simulink library "oceanFloorContactModel_ul"  (R2020a)
settings: Solver=VariableStepAuto  StartTime=0.0  StopTime=10.0  RelTol=1e-3
undefined symbols (not defined in the file): gndStn
libraries: vrlib x3, eulAng2RotMat_ul x1
settings Model: Creator=mitch  LastModifiedBy=mitch

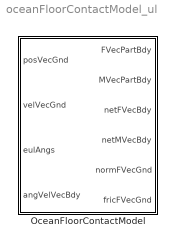
== system oceanFloorContactModel_ul ==
  OceanFloorContactModel : Subsystem  TreatAsAtomicUnit=on  mask{gs=gndStn, momArms=0}
      mask prompts: gs "OCT.floor ocean floor obj"; momArms "Vechicle moment arms"

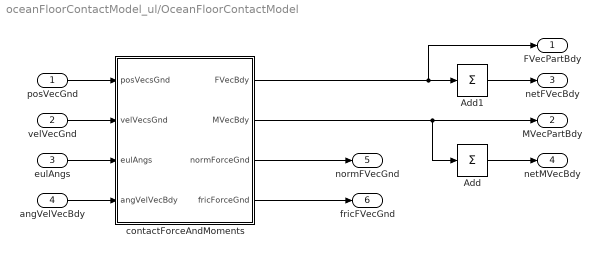
== system oceanFloorContactModel_ul/OceanFloorContactModel ==
  posVecGnd : Inport
  velVecGnd : Inport  Port=2
  eulAngs : Inport  Port=3
  angVelVecBdy : Inport  Port=4
  Add : Sum  Inputs=+  CollapseMode=Specified dimension  CollapseDim=2
  Add1 : Sum  Inputs=+  CollapseMode=Specified dimension  CollapseDim=2
  contactForceAndMoments : Subsystem  mask{z0=gs.bedrockZ.Value, z1=gs.oceanFloorZ.Value, zStar=gs.stiffnessZPt.Value, FStar=gs.stiffnessFMag.Value, mu=gs.fricCoeff.Value, momArmVecs=momArms}
      mask prompts: z0 "Bedrock z Position"; z1 "Ocean floor z Position"; zStar "Stiffness z Point"; FStar "Stiffness Normal Force [N]"; mu "Friction Coeff"; momArmVecs "Mom Arm Vecs Bdy"
  FVecPartBdy : Outport
  MVecPartBdy : Outport  Port=2
  netFVecBdy : Outport  Port=3
  netMVecBdy : Outport  Port=4
  normFVecGnd : Outport  Port=5
  fricFVecGnd : Outport  Port=6
  wires:
  contactForceAndMoments/1(FVecBdy) -> FVecPartBdy/1, Add1/1
  Add/1 -> netMVecBdy/1
  Add1/1 -> netFVecBdy/1
  contactForceAndMoments/2(MVecBdy) -> Add/1, MVecPartBdy/1
  eulAngs/1 -> contactForceAndMoments/3(eulAngs)
  posVecGnd/1 -> contactForceAndMoments/1(posVecsGnd)
  velVecGnd/1 -> contactForceAndMoments/2(velVecsGnd)
  angVelVecBdy/1 -> contactForceAndMoments/4(angVelVecBdy)
  contactForceAndMoments/3(normForceGnd) -> normFVecGnd/1
  contactForceAndMoments/4(fricForceGnd) -> fricFVecGnd/1

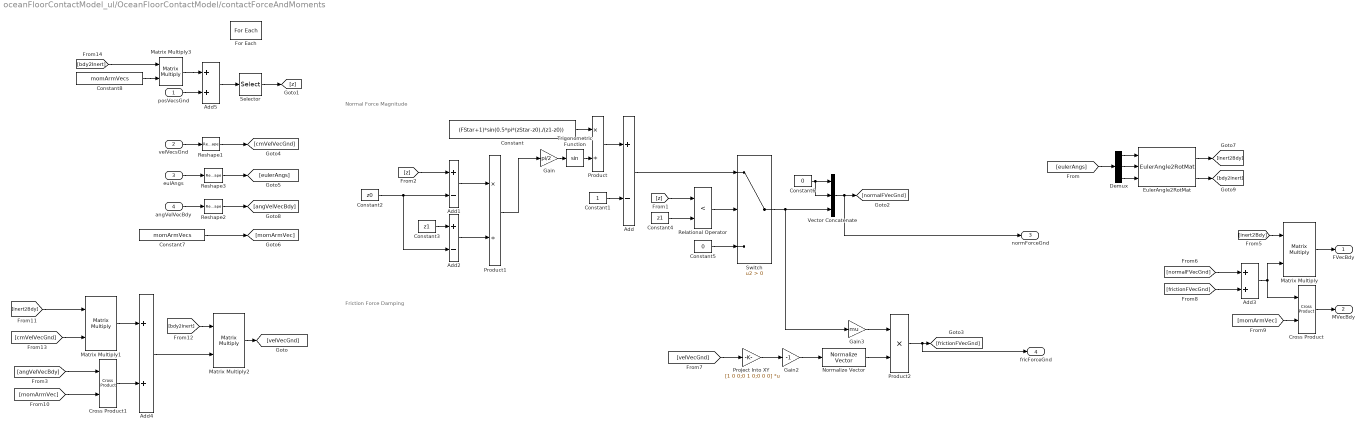
== system oceanFloorContactModel_ul/OceanFloorContactModel/contactForceAndMoments ==
  note: Friction Force Damping
  note: Normal Force Magnitude
  posVecsGnd : Inport  PortDimensions=[3 1]
  velVecsGnd : Inport  Port=2  PortDimensions=[3 1]
  eulAngs : Inport  Port=3  PortDimensions=[3 1]
  angVelVecBdy : Inport  Port=4  PortDimensions=[3 1]
  Add : Sum  Inputs=+-
  Add1 : Sum  Inputs=+-
  Add2 : Sum  Inputs=+-
  Add3 : Sum
  Add4 : Sum
  Add5 : Sum
  Constant : Constant  Value=(FStar+1)*sin(0.5*pi*(zStar-z0)./(z1-z0))
  Constant1 : Constant
  Constant2 : Constant  Value=z0
  Constant3 : Constant  Value=z1
  Constant4 : Constant  Value=z1
  Constant5 : Constant  Value=0
  Constant6 : Constant  Value=0
  Constant7 : Constant  Value=momArmVecs
  Constant8 : Constant  Value=momArmVecs
  Cross Product : vrlib/Utilities/Cross Product
  Cross Product1 : vrlib/Utilities/Cross Product
  Demux : Demux  Outputs=3
  EulerAngle2RotMat : eulAng2RotMat_ul/EulerAngle2RotMat  SystemSampleTime=-1  Latency=0  AutoFrameSizeCalculation=off
  For Each : ForEach  DisableCoverage=on  IterateSubsysMaskParameter=off,off,off,off,off,on  SubsysMaskParameterIterationDimension=1,1,1,1,1,2
  Gain : Gain  Gain=pi/2
  Gain2 : Gain  Gain=-1
  Gain3 : Gain  Gain=mu
  Matrix Multiply{,1..3} (4 alike) : Product  Multiplication=Matrix(*)
  Normalize Vector : vrlib/Utilities/Normalize Vector  maxzero=0
  Product : Product  Inputs=*/
  Product1 : Product  Inputs=*/
  Product2 : Product
  Project Into XY : Gain  Gain=[1 0 0;0 1 0;0 0 0]  Multiplication=Matrix(K*u)
  Relational Operator : RelationalOperator  Operator=<  OutDataTypeStr=boolean  RndMeth=Simplest
  Reshape1 : Reshape  OutputDimensionality=Column vector (2-D)
  Reshape2 : Reshape  OutputDimensionality=Column vector (2-D)
  Reshape3 : Reshape  OutputDimensionality=Column vector (2-D)
  Selector : Selector  InputPortWidth=3  IndexOptions=Index vector (dialog)  Indices=3  OutputSizes=1
  Switch : Switch  Criteria=u2 > Threshold
  Trigonometric Function : Trigonometry
  Vector Concatenate : Concatenate  NumInputs=3
  FVecBdy : Outport  ConcatenationDimension=2
  MVecBdy : Outport  Port=2  ConcatenationDimension=2
  normForceGnd : Outport  Port=3  ConcatenationDimension=2
  fricForceGnd : Outport  Port=4  ConcatenationDimension=2
  wires:
  Constant/1 -> Product/1
  posVecsGnd/1 -> Add5/2
  Product/1 -> Add/1
  Constant1/1 -> Add/2
  Trigonometric Function/1 -> Product/2
  Gain/1 -> Trigonometric Function/1
  Add1/1 -> Product1/1
  Add2/1 -> Product1/2
  Selector/1 -> [z]
  Constant2/1 -> Add2/2, Add1/2
  Constant3/1 -> Add2/1
  Product1/1 -> Gain/1
  Add/1 -> Switch/1
  [z] -> Relational Operator/1
  Constant4/1 -> Relational Operator/2
  Relational Operator/1 -> Switch/2
  [z] -> Add1/1
  Constant5/1 -> Switch/3
  velVecsGnd/1 -> Reshape1/1
  Project Into XY/1 -> Gain2/1
  Gain2/1 -> Normalize Vector/1
  Switch/1 -> Gain3/1, Vector Concatenate/3
  Gain3/1 -> Product2/1
  Normalize Vector/1 -> Product2/2
  Product2/1 -> fricForceGnd/1, [frictionFVecGnd]
  Reshape1/1 -> [cmVelVecGnd]
  [velVecGnd] -> Project Into XY/1
  Constant6/1 -> Vector Concatenate/2, Vector Concatenate/1
  eulAngs/1 -> Reshape3/1
  [eulerAngs] -> Demux/1
  Demux/1 -> EulerAngle2RotMat/1
  Demux/2 -> EulerAngle2RotMat/2
  Demux/3 -> EulerAngle2RotMat/3
  EulerAngle2RotMat/2 -> [bdy2Inert]
  EulerAngle2RotMat/1 -> [inert2Bdy]
  [normalFVecGnd] -> Add3/1
  [frictionFVecGnd] -> Add3/2
  Add3/1 -> Matrix Multiply/2, Cross Product/1
  Matrix Multiply/1 -> FVecBdy/1
  [inert2Bdy] -> Matrix Multiply/1
  Cross Product/1 -> MVecBdy/1
  [momArmVec] -> Cross Product/2
  Constant7/1 -> [momArmVec]
  angVelVecBdy/1 -> Reshape2/1
  Reshape2/1 -> [angVelVecBdy]
  Reshape3/1 -> [eulerAngs]
  [angVelVecBdy] -> Cross Product1/1
  [momArmVec] -> Cross Product1/2
  Cross Product1/1 -> Add4/2
  Add4/1 -> Matrix Multiply2/2
  [cmVelVecGnd] -> Matrix Multiply1/2
  [inert2Bdy] -> Matrix Multiply1/1
  Matrix Multiply1/1 -> Add4/1
  Matrix Multiply2/1 -> [velVecGnd]
  [bdy2Inert] -> Matrix Multiply2/1
  Vector Concatenate/1 -> normForceGnd/1, [normalFVecGnd]
  Add5/1 -> Selector/1
  Matrix Multiply3/1 -> Add5/1
  Constant8/1 -> Matrix Multiply3/2
  [bdy2Inert] -> Matrix Multiply3/1
